simulink model "Problem_2_Simulink"  (R2023a)
settings: Solver=VariableStepAuto  StartTime=0.0  StopTime=10.0  RelTol=1e-3
settings Model: Creator=eliasoa  LastModifiedBy=eliasoa

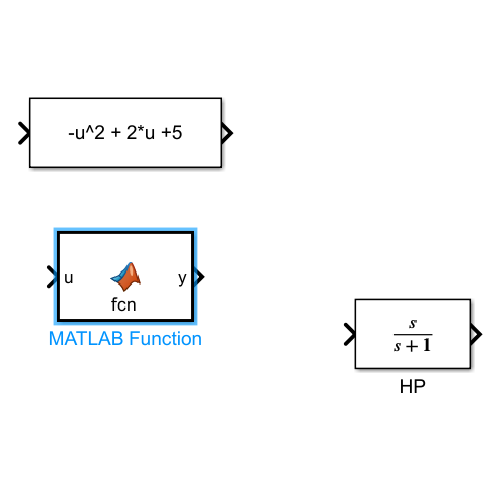
[thumbnail: Simulink's stored preview of the top-level diagram]
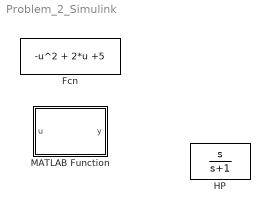
== system Problem_2_Simulink ==
  Fcn : Fcn  Expr=-u^2 + 2*u +5
  HP : TransferFcn  Numerator=[1 0]  Denominator=[1 1]
  MATLAB Function : MATLAB Function  TreatAsAtomicUnit=on

== matlab function Problem_2_Simulink/MATLAB Function ==
  data: u input; y output
function y = fcn(u)
y = -u^2 + 2 * u + 5;
